simulink model "smith_predictor"  (R2019a)
settings: Solver=FixedStepAuto  StartTime=0.0  StopTime=endtime  FixedStep=0.001  RelTol=1e-3
undefined symbols (not defined in the file or in its folder): Discrete, Gpd, K, R, Time
libraries: ctrlSharedLib x1
settings Model: Creator=chris  LastModifiedBy=chris

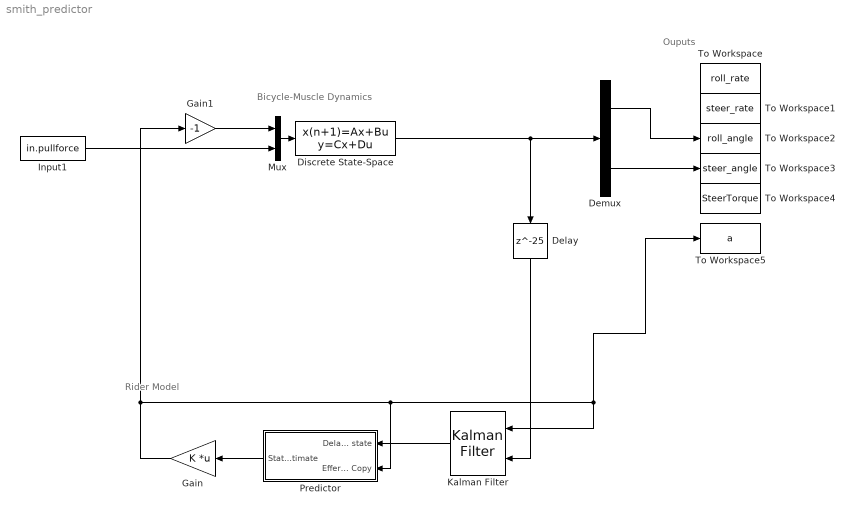
== system smith_predictor ==
  note: Rider Model
  note: Ouputs
  note: Bicycle-Muscle Dynamics
  Delay : Delay  DelayLength=25  InitialCondition=0
  Demux : Demux  Outputs=2
  Discrete State-Space : DiscreteStateSpace  A=Gpd.A  B=Gpd.B  C=Gpd.C  D=Gpd.D  SampleTime=-1
  Gain : Gain  Gain=K  Multiplication=Matrix(K*u) (u vector)
  Gain1 : Gain  Gain=-1
  Input1 : FromWorkspace  VariableName=in.pullforce  SampleTime=0
  Kalman Filter : ctrlSharedLib/Kalman Filter  TimeDomain=Discrete-Time  UseCurrentEstimator=on  ModelSource=Individual A, B, C, D matrices  ModelSourceVariable=ss(0.95,1,1,0,1)  A=Gpd.A  B=Gpd.B(:,1)  C=Gpd.C  D=Gpd.D(:,1)  NumberOfStates=1  NumberOfInputs=1  NumberOfOutputs=1  InitialEstimateSource=Dialog  X0=0  P0=10  UseK=off  UseGH=off  NumberOfProcessNoiseInputs=1  G=1  TimeInvariantG=on  H=0  TimeInvariantH=on  Q=Q  TimeInvariantQ=on  R=R  TimeInvariantR=on  N=0  TimeInvariantN=on  AddInputPort=on  AddEnablePort=off  OutputEstimatedY=off  OutputP=off  Ts=-1
      settings: SourceProductBaseCode=CT
  Mux : Mux  Inputs=2
  "Predictor " : Subsystem
  To Workspace : ToWorkspace  VariableName=roll_rate  SampleTime=-1
  To Workspace1 : ToWorkspace  VariableName=steer_rate  SampleTime=-1
  To Workspace2 : ToWorkspace  VariableName=roll_angle  SampleTime=-1
  To Workspace3 : ToWorkspace  VariableName=steer_angle  SampleTime=-1
  To Workspace4 : ToWorkspace  VariableName=SteerTorque  SampleTime=-1
  To Workspace5 : ToWorkspace  VariableName=a  SampleTime=-1
  wires:
  Discrete State-Space/1 -> Delay/1, Demux/1
  Delay/1 -> Kalman Filter/2
  Input1/1 -> Mux/2
  Demux/2 -> To Workspace3/1
  Gain/1 -> "Predictor "/2("Efference Copy "), Kalman Filter/1, To Workspace5/1, Gain1/1
  Demux/1 -> To Workspace2/1
  Mux/1 -> Discrete State-Space/1
  Kalman Filter/1 -> "Predictor "/1("Delayed state ")
  "Predictor "/1("State Estimate ") -> Gain/1
  Gain1/1 -> Mux/1

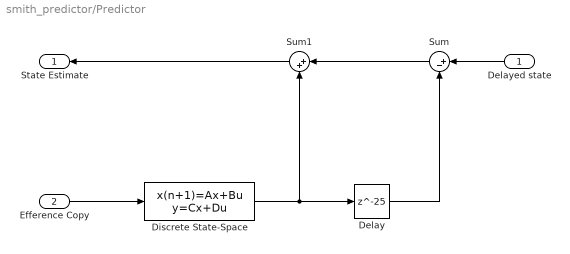
== system smith_predictor/Predictor  ==
  "Delayed state " : Inport
  "Efference Copy " : Inport  Port=2
  Delay : Delay  DelayLength=25  InitialCondition=0
  Discrete State-Space : DiscreteStateSpace  A=Gpd.A  B=Gpd.B(:,1)  C=Gpd.C  D=Gpd.D(:,1)  SampleTime=-1
  Sum : Sum  Inputs=|+-
  Sum1 : Sum  Inputs=|++
  "State Estimate " : Outport
  wires:
  "Efference Copy "/1 -> Discrete State-Space/1
  Delay/1 -> Sum/2
  "Delayed state "/1 -> Sum/1
  Sum/1 -> Sum1/1
  Discrete State-Space/1 -> Sum1/2, Delay/1
  Sum1/1 -> "State Estimate "/1
